simulink model "sf_msg_data_syntax_and_lifetime"  (R2017b)
settings: Solver=FixedStepDiscrete  StartTime=0.0  StopTime=10.0  FixedStep=1  RelTol=1e-3  EnableMultiTasking=on
settings Model: Creator=The MathWorks, Inc.  LastModifiedBy=The MathWorks, Inc.
settings DataIOCC: LimitDataPoints=on  SaveFormat=Array
settings OptimizationCC: ExpressionDepthLimit=2147483647  LifeSpan=1
settings DebuggingCC: UnderspecifiedInitializationDetection=Classic  MergeDetectMultiDrivingBlocksExec=none  SolverPrmCheckMsg=warning  AllowSymbolicDim=off  StateNameClashWarn=warning  SFUnexpectedBacktrackingDiag=warning  SFNoUnconditionalDefaultTransitionDiag=warning  SFExecutionAtInitializationDiag=none
settings HardwareCC: ProdBitPerPointer=32  ProdBitPerSizeT=32  ProdBitPerPtrDiffT=32  ProdLargestAtomicFloat=None  ProdIntDivRoundTo=Undefined  ProdEndianess=Unspecified  ProdWordSize=32  ProdHWDeviceType=32-bit Generic
settings ModelReferenceCC: PropagateSignalLabelsOutOfModel=off
settings SFSimCC: MATLABDynamicMemAlloc=off
settings RTWCC: SystemTargetFile=ert.tlc  TemplateMakefile=ert_default_tmf  Description=Real-Time Workshop Embedded Coder
settings CodeAppCC: IgnoreCustomStorageClasses=off  CustomSymbolStrType=$N$R$M  StateflowObjectComments=on  InternalIdentifier=Classic
settings ERTTargetCC: MultiwordLength=2048  GenerateSampleERTMain=on  ERTCustomFileTemplate=example_file_process.tlc  ConvertIfToSwitch=off  SuppressUnreachableDefaultCases=off
settings ConfigComp: CovMetricSettings=dw  CovHtmlReporting=on  CovSaveCumulativeToWorkspaceVar=on  CovSaveSingleToWorkspaceVar=on  CovExternalEMLEnable=off  CovSFcnEnable=off

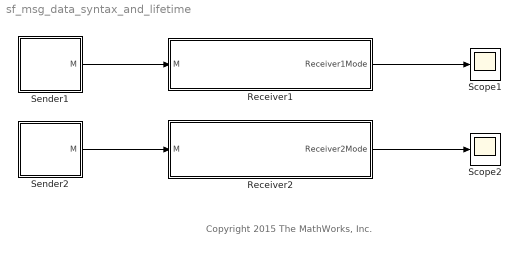
== system sf_msg_data_syntax_and_lifetime ==
  note: Copyright 2015 The MathWorks, Inc.
  Receiver1 : Stateflow chart  TreatAsAtomicUnit=on
  Receiver2 : Stateflow chart  TreatAsAtomicUnit=on
  Scope1 : Scope
  Scope2 : Scope
  Sender1 : Stateflow chart  TreatAsAtomicUnit=on
  Sender2 : Stateflow chart  TreatAsAtomicUnit=on
  wires:
  Sender2/1(M) -> Receiver2/1(M)
  Receiver2/1(Receiver2Mode) -> Scope2/1
  Sender1/1(M) -> Receiver1/1(M)
  Receiver1/1(Receiver1Mode) -> Scope1/1

== stateflow chart sf_msg_data_syntax_and_lifetime/Sender2 ==
  state A
    en:
    M.data = 3;
    send(M);
    M.data = 5;
    send(M);
  (default) -> A
  data: M output double

== stateflow chart sf_msg_data_syntax_and_lifetime/Receiver2 ==
  state B
    state B1
    state B2
    (default) -> (junction 21)
    (junction 21) -> B1 [order 1] : M[M.data == 3]
    (junction 21) -> (junction 24) [order 2]
    (junction 24) -> B2
  state A
  (default) -> A
  A -> B : M
  data: M input double; Receiver2Mode output Enum: Receiver2ModeType

== stateflow chart sf_msg_data_syntax_and_lifetime/Receiver1 ==
  state A
  state B
  (default) -> A
  A -> B : M[M.data == 5]
  data: M input double; Receiver1Mode output Enum: Receiver1ModeType

== stateflow chart sf_msg_data_syntax_and_lifetime/Sender1 ==
  state A
    en:
    M.data = 3;
    send(M);
  state B
    en:
    M.data = 5;
    send(M);
  (default) -> A
  A -> B : after(3,sec)
  data: M output double
